simulink model "sampleModel168"  (R2021b)
settings: Solver=VariableStepAuto  StartTime=0.0  StopTime=10.0  RelTol=1e-3
undefined symbols (not defined in the file or in its folder): DiscIntNeverNeededParam
libraries: simulink x10, slpidlib x2
settings Model: Creator=user  LastModifiedBy=user

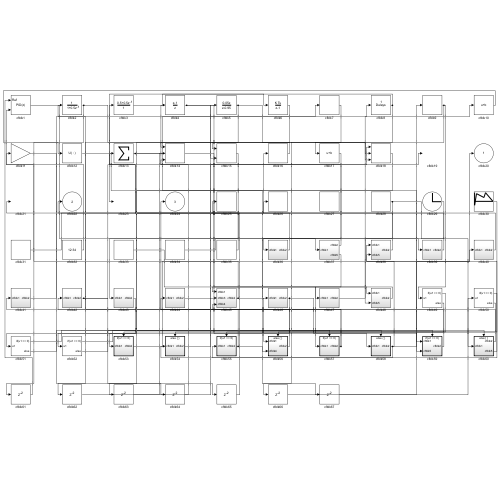
[thumbnail: Simulink's stored preview of the top-level diagram]
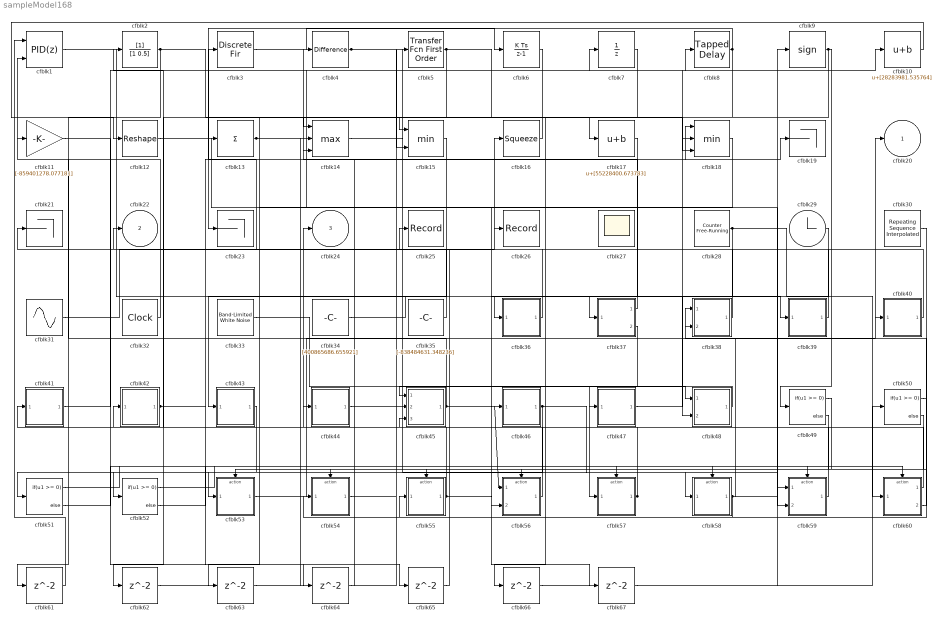
== system sampleModel168 ==
  cfblk1 : slpidlib/PID Controller (2DOF)  Controller=PID  Form=Parallel  TimeDomain=Discrete-time  UseExternalTs=off  SampleTime=1  IntegratorMethod=Forward Euler  FilterMethod=Forward Euler  ControllerParametersSource=internal  P=1  I=1  D=0  UseFilter=on  N=100  b=1  c=1  TunerSelectOption=Transfer Function Based (PID Tuner App)  InitialConditionSource=internal  InitialConditionForIntegrator=0  InitialConditionForFilter=0  DifferentiatorICPrevScaledInput=0  ExternalReset=none  TrackingMode=off  Kt=1  LimitOutput=off  SatLimitsSource=internal  UpperSaturationLimit=inf  LowerSaturationLimit=-inf  LinearizeAsGain=off  AntiWindupMode=none  Kb=1  POutMin=[]  POutMax=[]  IOutMin=[]  IOutMax=[]  DOutMin=[]  DOutMax=[]  NOutMin=[]  NOutMax=[]  bOutMin=[]  bOutMax=[]  cOutMin=[]  cOutMax=[]  SumOutMin=[]  SumOutMax=[]  SaturationOutMin=[]  SaturationOutMax=[]  PParamMin=[]  PParamMax=[]  IParamMin=[]  IParamMax=[]  DParamMin=[]  DParamMax=[]  NParamMin=[]  NParamMax=[]  bParamMin=[]  bParamMax=[]  cParamMin=[]  cParamMax=[]  KbParamMin=[]  KbParamMax=[]  KtParamMin=[]  KtParamMax=[]  KbOutMin=[]  KbOutMax=[]  KtOutMin=[]  KtOutMax=[]  IntegratorOutMin=[]  IntegratorOutMax=[]  FilterOutMin=[]  FilterOutMax=[]  SumI1OutMin=[]  SumI1OutMax=[]  SumI2OutMin=[]  SumI2OutMax=[]  SumI3OutMin=[]  SumI3OutMax=[]  SumI4OutMin=[]  SumI4OutMax=[]  SumDOutMin=[]  SumDOutMax=[]  Sum1OutMin=[]  Sum1OutMax=[]  Sum2OutMin=[]  Sum2OutMax=[]  Sum3OutMin=[]  Sum3OutMax=[]  DifferentiatorOutMin=[]  DifferentiatorOutMax=[]  FilterDiffOutCoefMin=[]  FilterDiffOutCoefMax=[]  ReciprocalOutMin=[]  ReciprocalOutMax=[]  SumDenOutMin=[]  SumDenOutMax=[]  SumNumOutMin=[]  SumNumOutMax=[]  DivideOutMin=[]  DivideOutMax=[]  UdiffTsProdOutMin=[]  UdiffTsProdOutMax=[]  NTsProdOutMin=[]  NTsProdOutMax=[]  UintegralTsProdOutMin=[]  UintegralTsProdOutMax=[]  UngainTsProdOutMin=[]  UngainTsProdOutMax=[]  IntegratorContinuousStateAttributes=''  IntegratorStateMustResolveToSignalObject=off  IntegratorRTWStateStorageClass=Auto  FilterContinuousStateAttributes=''  FilterStateMustResolveToSignalObject=off  FilterRTWStateStorageClass=Auto  ParallelPVariant=InternalParameters  IdealPVariant=Disabled  IVariant=InternalParameters  DVariant=InternalParameters  bVariant=InternalParameters  cVariant=InternalParameters  IntegratorVariant=Discrete  SatVariant=Disabled  AWVariant=Passthrough  PCopyVariant=Disabled  TRVariant=Disabled  FdbkBlocksVariant=Forward  IdealPFdbkVariant=Disabled  SatFdbkVariant=Disabled  DerivativeFilterVariant=ForwardEulerFilter  NVariant=InternalParameters  NCopyVariant=Disabled  FilterICVariant=InternalICsFilter  IntegratorICVariant=InternalICs  ExternalResetVariant=Disabled  TRSumVariant=Passthrough  SumFdbkVariant=Disabled  SumVariant=Sum_PID  TsampFilterVariant=InternalTs  TsampNgainVariant=Passthrough  TsampIntegralVariant=Passthrough  ExternalSaturationOutDataTypeStr=Inherit: Same as second input
      settings: SourceProductBaseCode=SL
  cfblk10 : Bias  Bias=[28283981.535764]
  cfblk11 : Gain  Gain=[-859401278.077181]
  cfblk12 : Reshape
  cfblk13 : Sum  Inputs=+
  cfblk14 : MinMax  Function=max  Inputs=3
  cfblk15 : MinMax  Inputs=2
  cfblk16 : Squeeze
  cfblk17 : Bias  Bias=[55228400.673783]
  cfblk18 : MinMax  Inputs=3
  cfblk19 : Terminator
  cfblk2 : DiscreteFilter  SampleTime=1
  cfblk21 : Terminator
  cfblk23 : Terminator
  cfblk25 : Record  FileSettingsInternal="{\"entries\":[{\"content\":{\"excelSettings\":{\"content\":{},\"type\":\"Streamout.ExcelSettings\"}},\"type\":\"Streamout.FileSettingStorage\",\"uuid\":\"5d6700eb-b7dc-4e89-8cfd-a7cfabde85fd\"}],\"packageUris\":[\"http://schema.mathworks.com/mf0/streamout_blocks/R2020a\"],\"version\":\"1.0\"}"  SignalsInternal="{\"entries\":[{\"content\":{\"signals\":[{\"content\":{\"blockPath\":[\"sampleModel168/cfblk25\"],\"channel\":[],\"dimensions\":[1],\"domain\":\"sampleModel168/cfblk25\",\"lineColor\":\"#ff13a6\",\"plots\":[1],\"port\":1,\"sid\":[\"\"],\"signalID\":6325,\"signalName\":\"cfblk57\"},\"type\":\"RecordBlkView.Signal\",\"uuid\":\"5bee3f64-e3fd-44b3-9e31-3812ad4f074b\"}]},\"type\":\"RecordBlkView.InputSignals\",\"uuid\":\"565ec13a-f817-448c-bf93-5228326c90da\"}],\"packageUris\":[\"http://schema.mathworks.com/mf0/streamout_blocks/R2020a\"],\"version\":\"1.0\"}"  VisualizationBindings="{\"sparklinesplugin\":{\"info\":[{\"bindingParametersList\":[],\"subplotID\":1}]}}"
  cfblk26 : Record  FileSettingsInternal="{\"entries\":[{\"content\":{\"excelSettings\":{\"content\":{},\"type\":\"Streamout.ExcelSettings\"}},\"type\":\"Streamout.FileSettingStorage\",\"uuid\":\"034f7d33-27da-4be1-a58b-e2f12ee0a9b7\"}],\"packageUris\":[\"http://schema.mathworks.com/mf0/streamout_blocks/R2020a\"],\"version\":\"1.0\"}"  SignalsInternal="{\"entries\":[{\"content\":{\"signals\":[{\"content\":{\"blockPath\":[\"sampleModel168/cfblk26\"],\"channel\":[],\"dimensions\":[1],\"domain\":\"sampleModel168/cfblk26\",\"lineColor\":\"#fe330a\",\"plots\":[1],\"port\":1,\"sid\":[\"\"],\"signalID\":6329,\"signalName\":\"cfblk31\"},\"type\":\"RecordBlkView.Signal\",\"uuid\":\"832ba97a-a374-4f23-ac50-8a6ca30bdff1\"}]},\"type\":\"RecordBlkView.InputSignals\",\"uuid\":\"b795735d-caf7-44f9-b6f9-1499413fef97\"}],\"packageUris\":[\"http://schema.mathworks.com/mf0/streamout_blocks/R2020a\"],\"version\":\"1.0\"}"  VisualizationBindings="{\"sparklinesplugin\":{\"info\":[{\"bindingParametersList\":[],\"subplotID\":1}]}}"
  cfblk27 : Scope
      settings: Floating=on
  cfblk28 : simulink/Sources/Counter Free-Running  NumBits=[13.000000]  tsamp=-1
  cfblk29 : Clock
  cfblk3 : DiscreteFir  SampleTime=1
  cfblk30 : simulink/Sources/Repeating Sequence Interpolated  OutValues=[-245595446.303233, 532111753.343580, 271370774.628076, 605929342.259745, 14003262.711225]  TimeValues=[0 0.1 0.5 0.6 1].'  LookUpMeth=Interpolation-Use End Values  tsamp=0.01  OutMin=[]  OutMax=[]  OutDataTypeStr=double  OutputDataTypeScalingMode=double  OutDataType=fixdt(0,8)  OutScaling=2^-10
  cfblk31 : Sin  Amplitude=[-188151696.405672]  Bias=[-383980109.260124]  SampleTime=0
  cfblk32 : DigitalClock
  cfblk33 : simulink/Sources/Band-Limited White Noise  Cov=[8926345468.360197]  Ts=0.1  seed=[3976395025.000000]
  cfblk34 : Constant  Value=[400865686.655921]  SampleTime=1
  cfblk35 : Constant  Value=[-838484631.348236]  SampleTime=1
  cfblk36 : Subsystem
  cfblk37 : Subsystem
  cfblk38 : Subsystem
  cfblk39 : Subsystem
  cfblk4 : simulink/Discrete/Difference  ICPrevInput=0.0  OutMin=[]  OutMax=[]  OutDataTypeStr=Inherit: Inherit via back propagation  OutDataType=fixdt(1, 16)  OutScaling=2^-10  DoSatur=off
  cfblk40 : Subsystem
  cfblk41 : Subsystem
  cfblk42 : Subsystem
  cfblk43 : Subsystem
  cfblk44 : Subsystem
  cfblk45 : Subsystem
  cfblk46 : Subsystem
  cfblk47 : Subsystem
  cfblk48 : Subsystem
  cfblk{49..52} (4 alike) : If  IfExpression=u1 >= 0  SampleTime=1
  cfblk5 : simulink/Discrete/Transfer Fcn First Order  PoleZ=0.95  ICPrevOutput=0.0  DoSatur=off
  cfblk53 : Subsystem  TreatAsAtomicUnit=on
  cfblk54 : Subsystem  TreatAsAtomicUnit=on
  cfblk55 : Subsystem  TreatAsAtomicUnit=on
  cfblk56 : Subsystem  TreatAsAtomicUnit=on
  cfblk57 : Subsystem  TreatAsAtomicUnit=on
  cfblk58 : Subsystem  TreatAsAtomicUnit=on
  cfblk59 : Subsystem  TreatAsAtomicUnit=on
  cfblk6 : DiscreteIntegrator  ICPrevOutput=DiscIntNeverNeededParam  ICPrevScaledInput=DiscIntNeverNeededParam
  cfblk60 : Subsystem  TreatAsAtomicUnit=on
  cfblk{61..67} (7 alike) : Delay  SampleTime=1
  cfblk7 : UnitDelay  HasFrameUpgradeWarning=on
  cfblk8 : simulink/Discrete/Tapped Delay  vinit=0.0  samptime=-1  NumDelays=1  DelayOrder=Oldest  includeCurrent=off
  cfblk9 : Signum
  cfblk20 : Outport
  cfblk22 : Outport  Port=2
  cfblk24 : Outport  Port=3
  wires:
  cfblk39/1(cfblk2) -> cfblk16/1
  cfblk2/1 -> cfblk15/2, cfblk61/1
  cfblk53/1(cfblk2) -> cfblk20/1
  cfblk1/1 -> cfblk39/1(cfblk1)
  cfblk55/1(cfblk2) -> cfblk44/1(cfblk1), cfblk67/1
  cfblk14/1 -> cfblk48/1(cfblk1)
  cfblk4/1 -> cfblk58/1(cfblk1), cfblk18/3
  cfblk10/1 -> cfblk12/1
  cfblk8/1 -> cfblk23/1, cfblk63/1
  cfblk29/1 -> cfblk48/2(cfblk5)
  cfblk9/1 -> cfblk49/1, cfblk17/1
  cfblk31/1 -> cfblk26/1
  cfblk43/1(cfblk2) -> cfblk51/1
  cfblk48/1(cfblk2) -> cfblk45/1(cfblk1)
  cfblk30/1 -> cfblk55/1(cfblk1)
  cfblk46/1(cfblk2) -> cfblk52/1, cfblk59/2(cfblk5)
  cfblk34/1 -> cfblk37/1(cfblk1)
  cfblk59/1(cfblk2) -> cfblk42/1(cfblk1)
  cfblk45/1(cfblk2) -> cfblk56/1(cfblk1), cfblk11/1
  cfblk15/1 -> cfblk43/1(cfblk1)
  cfblk12/1 -> cfblk46/1(cfblk1)
  cfblk28/1 -> cfblk56/2(cfblk4), cfblk60/1(cfblk1)
  cfblk44/1(cfblk2) -> cfblk5/1
  cfblk38/1(cfblk2) -> cfblk3/1
  cfblk7/1 -> cfblk36/1(cfblk1)
  cfblk60/1(cfblk2) -> cfblk24/1
  cfblk3/1 -> cfblk6/1
  cfblk32/1 -> cfblk1/2
  cfblk60/2(cfblk5) -> cfblk38/1(cfblk1)
  cfblk40/1(cfblk2) -> cfblk13/1
  cfblk36/1(cfblk2) -> cfblk22/1
  cfblk13/1 -> cfblk8/1, cfblk59/1(cfblk1)
  cfblk35/1 -> cfblk21/1
  cfblk54/1(cfblk2) -> cfblk19/1
  cfblk42/1(cfblk2) -> cfblk18/1, cfblk64/1
  cfblk18/1 -> cfblk53/1(cfblk1)
  cfblk58/1(cfblk2) -> cfblk38/2(cfblk5), cfblk40/1(cfblk1), cfblk54/1(cfblk1)
  cfblk37/1(cfblk2) -> cfblk4/1
  cfblk33/1 -> cfblk57/1(cfblk1)
  cfblk57/1(cfblk2) -> cfblk25/1, cfblk41/1(cfblk1)
  cfblk41/1(cfblk2) -> cfblk7/1
  cfblk16/1 -> cfblk14/1
  cfblk56/1(cfblk2) -> cfblk2/1
  cfblk37/2(cfblk5) -> cfblk47/1(cfblk1)
  cfblk47/1(cfblk2) -> cfblk10/1
  cfblk5/1 -> cfblk18/2, cfblk15/1
  cfblk49/1 -> cfblk53/Action
  cfblk49/2 -> cfblk54/Action
  cfblk50/1 -> cfblk55/Action
  cfblk50/2 -> cfblk56/Action
  cfblk51/1 -> cfblk57/Action
  cfblk51/2 -> cfblk58/Action
  cfblk52/1 -> cfblk59/Action
  cfblk52/2 -> cfblk60/Action
  cfblk61/1 -> cfblk1/1
  cfblk6/1 -> cfblk62/1
  cfblk62/1 -> cfblk45/2(cfblk3)
  cfblk63/1 -> cfblk14/2
  cfblk64/1 -> cfblk14/3
  cfblk11/1 -> cfblk65/1
  cfblk65/1 -> cfblk45/3(cfblk4)
  cfblk17/1 -> cfblk66/1
  cfblk66/1 -> cfblk9/1
  cfblk67/1 -> cfblk50/1

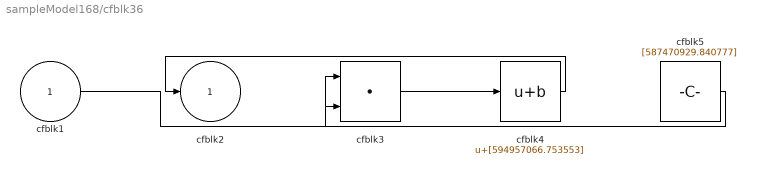
== system sampleModel168/cfblk36 ==
  cfblk1 : Inport
  cfblk3 : DotProduct  InputSameDT=on  OutDataTypeStr=Inherit: Inherit via internal rule
  cfblk4 : Bias  Bias=[594957066.753553]
  cfblk5 : Constant  Value=[587470929.840777]  SampleTime=1
  cfblk2 : Outport
  wires:
  cfblk4/1 -> cfblk2/1
  cfblk5/1 -> cfblk3/1
  cfblk1/1 -> cfblk3/2
  cfblk3/1 -> cfblk4/1

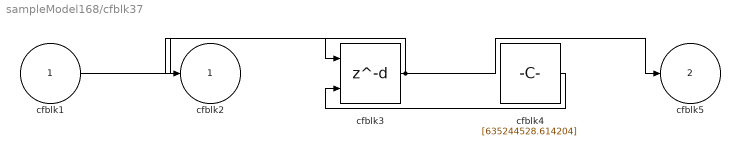
== system sampleModel168/cfblk37 ==
  cfblk1 : Inport
  cfblk3 : Delay  DelayLengthSource=Input port  SampleTime=1
      settings: InputPortMap=u0,p1
  cfblk4 : Constant  Value=[635244528.614204]  SampleTime=1
  cfblk2 : Outport
  cfblk5 : Outport  Port=2
  wires:
  cfblk1/1 -> cfblk3/1
  cfblk4/1 -> cfblk3/2
  cfblk3/1 -> cfblk5/1, cfblk2/1

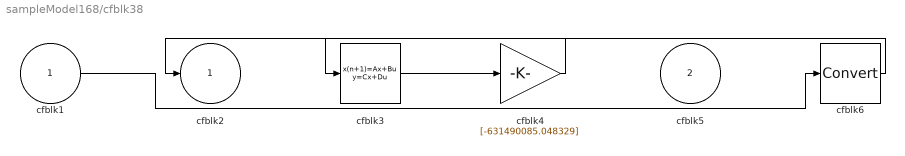
== system sampleModel168/cfblk38 ==
  cfblk1 : Inport
  cfblk5 : Inport  Port=2
  cfblk3 : DiscreteStateSpace
  cfblk4 : Gain  Gain=[-631490085.048329]
  cfblk6 : DataTypeConversion
  cfblk2 : Outport
  wires:
  cfblk4/1 -> cfblk2/1
  cfblk3/1 -> cfblk4/1
  cfblk1/1 -> cfblk6/1
  cfblk6/1 -> cfblk3/1

== system sampleModel168/cfblk39 ==
  cfblk1 : Inport
  cfblk3 : Delay  ShowEnablePort=on  SampleTime=1
      settings: InputPortMap=u0,e6
  cfblk4 : Product  Inputs=*
  cfblk2 : Outport
  wires:
  cfblk3/1 -> cfblk4/1
  cfblk4/1 -> cfblk2/1
  cfblk1/1 -> cfblk3/1, cfblk3/2

== system sampleModel168/cfblk40 ==
  cfblk1 : Inport
  cfblk3 : Assignment  DiagnosticForDimensions=Warning  IndexOptions=Index vector (dialog)  Indices=1  OutputSizes=1
  cfblk4 : Squeeze
  cfblk5 : Delay  SampleTime=1
  cfblk2 : Outport
  wires:
  cfblk1/1 -> cfblk2/1, cfblk3/2
  cfblk3/1 -> cfblk4/1
  cfblk4/1 -> cfblk5/1
  cfblk5/1 -> cfblk3/1

== system sampleModel168/cfblk41 ==
  cfblk1 : Inport
  cfblk3 : Constant  Value=[481463606.367237]  SampleTime=1
  cfblk2 : Outport
  wires:
  cfblk1/1 -> cfblk2/1

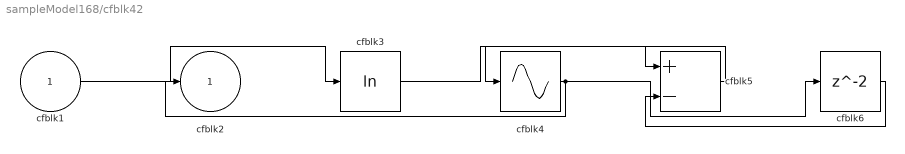
== system sampleModel168/cfblk42 ==
  cfblk1 : Inport
  cfblk3 : Math  Operator=log  SaturateOnIntegerOverflow=on
  cfblk4 : Sin  TimeSource=Use external signal  SampleTime=0
  cfblk5 : Sum  Inputs=+-
  cfblk6 : Delay  SampleTime=1
  cfblk2 : Outport
  wires:
  cfblk5/1 -> cfblk4/1
  cfblk1/1 -> cfblk3/1
  cfblk4/1 -> cfblk2/1, cfblk6/1
  cfblk3/1 -> cfblk5/1
  cfblk6/1 -> cfblk5/2

== system sampleModel168/cfblk43 ==
  cfblk1 : Inport
  cfblk3 : Sum
  cfblk4 : Sqrt  SaturateOnIntegerOverflow=on
  cfblk2 : Outport
  wires:
  cfblk4/1 -> cfblk2/1
  cfblk1/1 -> cfblk3/1, cfblk3/2
  cfblk3/1 -> cfblk4/1

== system sampleModel168/cfblk44 ==
  cfblk1 : Inport
  cfblk3 : DiscreteFilter  SampleTime=1
  cfblk2 : Outport
  wires:
  cfblk3/1 -> cfblk2/1
  cfblk1/1 -> cfblk3/1

== system sampleModel168/cfblk45 ==
  cfblk1 : Inport
  cfblk3 : Inport  Port=2
  cfblk4 : Inport  Port=3
  cfblk2 : Outport
  wires:
  cfblk3/1 -> cfblk2/1

== system sampleModel168/cfblk46 ==
  cfblk1 : Inport
  cfblk3 : Sum  Inputs=+-
  cfblk4 : Constant  Value=[-620973780.645703]  SampleTime=1
  cfblk2 : Outport
  wires:
  cfblk4/1 -> cfblk3/1
  cfblk1/1 -> cfblk3/2
  cfblk3/1 -> cfblk2/1

== system sampleModel168/cfblk47 ==
  cfblk1 : Inport
  cfblk3 : simulink/Discrete/Transfer Fcn Real Zero  ZeroZ=0.75  ICPrevInput=0.0  DoSatur=off
      settings: SourceProductBaseCode=SL
  cfblk4 : simulink/Discrete/Transfer Fcn Lead or Lag  PoleZ=0.95  ZeroZ=0.75  ICPrevOutput=0.0  ICPrevInput=0.0  DoSatur=off
      settings: SourceProductBaseCode=SL
  cfblk5 : simulink/Discrete/Transfer Fcn First Order  PoleZ=0.95  ICPrevOutput=0.0  DoSatur=off
  cfblk2 : Outport
  wires:
  cfblk1/1 -> cfblk5/1, cfblk3/1
  cfblk4/1 -> cfblk2/1
  cfblk5/1 -> cfblk4/1

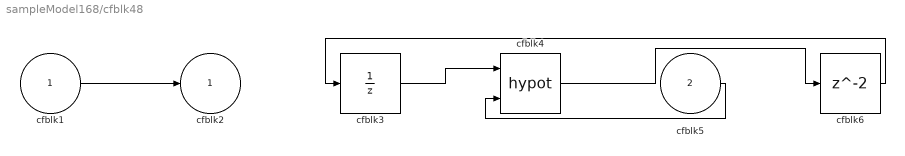
== system sampleModel168/cfblk48 ==
  cfblk1 : Inport
  cfblk5 : Inport  Port=2
  cfblk3 : UnitDelay  HasFrameUpgradeWarning=on
  cfblk4 : Math  Operator=hypot  SaturateOnIntegerOverflow=on
  cfblk6 : Delay  SampleTime=1
  cfblk2 : Outport
  wires:
  cfblk3/1 -> cfblk4/1
  cfblk1/1 -> cfblk2/1
  cfblk5/1 -> cfblk4/2
  cfblk4/1 -> cfblk6/1
  cfblk6/1 -> cfblk3/1

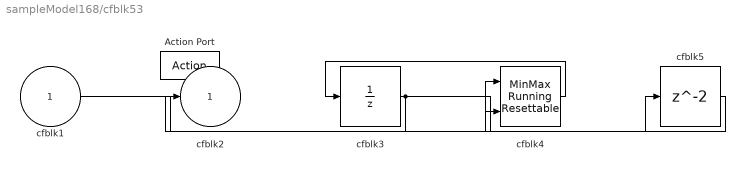
== system sampleModel168/cfblk53 ==
  cfblk1 : Inport
  Action Port : ActionPort  ActionPortLabel=if(u1 >= 0)
  cfblk3 : UnitDelay  SampleTime=-1  HasFrameUpgradeWarning=on
  cfblk4 : simulink/Math Operations/MinMax Running Resettable  Function=min  vinit=0.0
  cfblk5 : Delay
  cfblk2 : Outport
  wires:
  cfblk1/1 -> cfblk4/1
  cfblk4/1 -> cfblk3/1
  cfblk3/1 -> cfblk2/1, cfblk5/1
  cfblk5/1 -> cfblk4/2

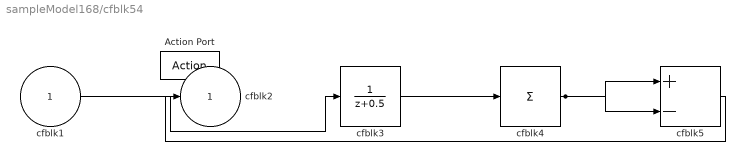
== system sampleModel168/cfblk54 ==
  cfblk1 : Inport
  Action Port : ActionPort  ActionPortLabel=else
  cfblk3 : DiscreteTransferFcn
  cfblk4 : Sum  Inputs=+
  cfblk5 : Sum  Inputs=+-
  cfblk2 : Outport
  wires:
  cfblk1/1 -> cfblk3/1
  cfblk5/1 -> cfblk2/1
  cfblk3/1 -> cfblk4/1
  cfblk4/1 -> cfblk5/1, cfblk5/2

== system sampleModel168/cfblk55 ==
  cfblk1 : Inport
  Action Port : ActionPort  ActionPortLabel=if(u1 >= 0)
  cfblk3 : Constant  Value=[634847590.051330]  SampleTime=1
  cfblk2 : Outport
  wires:
  cfblk1/1 -> cfblk2/1

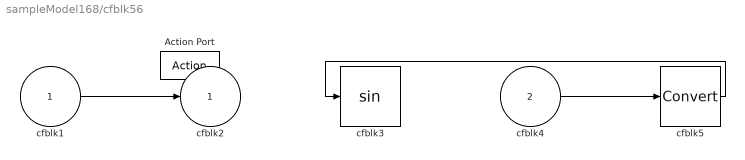
== system sampleModel168/cfblk56 ==
  cfblk1 : Inport
  cfblk4 : Inport  Port=2
  Action Port : ActionPort  ActionPortLabel=else
  cfblk3 : Trigonometry
  cfblk5 : DataTypeConversion
  cfblk2 : Outport
  wires:
  cfblk1/1 -> cfblk2/1
  cfblk4/1 -> cfblk5/1
  cfblk5/1 -> cfblk3/1

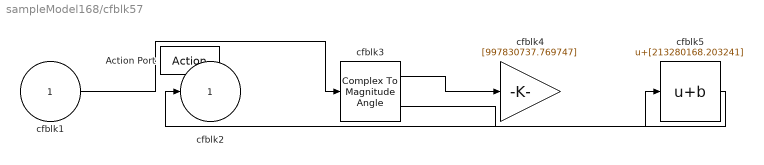
== system sampleModel168/cfblk57 ==
  cfblk1 : Inport
  Action Port : ActionPort  ActionPortLabel=if(u1 >= 0)
  cfblk3 : ComplexToMagnitudeAngle
  cfblk4 : Gain  Gain=[997830737.769747]
  cfblk5 : Bias  Bias=[213280168.203241]
  cfblk2 : Outport
  wires:
  cfblk5/1 -> cfblk2/1
  cfblk3/1 -> cfblk4/1
  cfblk3/2 -> cfblk5/1
  cfblk1/1 -> cfblk3/1

== system sampleModel168/cfblk58 ==
  cfblk1 : Inport
  Action Port : ActionPort  ActionPortLabel=else
  cfblk3 : slpidlib/PID Controller (2DOF)  Controller=PID  Form=Parallel  TimeDomain=Discrete-time  UseExternalTs=off  SampleTime=-1  IntegratorMethod=Forward Euler  FilterMethod=Forward Euler  ControllerParametersSource=internal  P=1  I=1  D=0  UseFilter=on  N=100  b=1  c=1  TunerSelectOption=Transfer Function Based (PID Tuner App)  InitialConditionSource=internal  InitialConditionForIntegrator=0  InitialConditionForFilter=0  DifferentiatorICPrevScaledInput=0  ExternalReset=none  TrackingMode=off  Kt=1  LimitOutput=off  SatLimitsSource=internal  UpperSaturationLimit=inf  LowerSaturationLimit=-inf  LinearizeAsGain=off  AntiWindupMode=none  Kb=1  POutMin=[]  POutMax=[]  IOutMin=[]  IOutMax=[]  DOutMin=[]  DOutMax=[]  NOutMin=[]  NOutMax=[]  bOutMin=[]  bOutMax=[]  cOutMin=[]  cOutMax=[]  SumOutMin=[]  SumOutMax=[]  SaturationOutMin=[]  SaturationOutMax=[]  PParamMin=[]  PParamMax=[]  IParamMin=[]  IParamMax=[]  DParamMin=[]  DParamMax=[]  NParamMin=[]  NParamMax=[]  bParamMin=[]  bParamMax=[]  cParamMin=[]  cParamMax=[]  KbParamMin=[]  KbParamMax=[]  KtParamMin=[]  KtParamMax=[]  KbOutMin=[]  KbOutMax=[]  KtOutMin=[]  KtOutMax=[]  IntegratorOutMin=[]  IntegratorOutMax=[]  FilterOutMin=[]  FilterOutMax=[]  SumI1OutMin=[]  SumI1OutMax=[]  SumI2OutMin=[]  SumI2OutMax=[]  SumI3OutMin=[]  SumI3OutMax=[]  SumI4OutMin=[]  SumI4OutMax=[]  SumDOutMin=[]  SumDOutMax=[]  Sum1OutMin=[]  Sum1OutMax=[]  Sum2OutMin=[]  Sum2OutMax=[]  Sum3OutMin=[]  Sum3OutMax=[]  DifferentiatorOutMin=[]  DifferentiatorOutMax=[]  FilterDiffOutCoefMin=[]  FilterDiffOutCoefMax=[]  ReciprocalOutMin=[]  ReciprocalOutMax=[]  SumDenOutMin=[]  SumDenOutMax=[]  SumNumOutMin=[]  SumNumOutMax=[]  DivideOutMin=[]  DivideOutMax=[]  UdiffTsProdOutMin=[]  UdiffTsProdOutMax=[]  NTsProdOutMin=[]  NTsProdOutMax=[]  UintegralTsProdOutMin=[]  UintegralTsProdOutMax=[]  UngainTsProdOutMin=[]  UngainTsProdOutMax=[]  IntegratorContinuousStateAttributes=''  IntegratorStateMustResolveToSignalObject=off  IntegratorRTWStateStorageClass=Auto  FilterContinuousStateAttributes=''  FilterStateMustResolveToSignalObject=off  FilterRTWStateStorageClass=Auto  ParallelPVariant=InternalParameters  IdealPVariant=Disabled  IVariant=InternalParameters  DVariant=InternalParameters  bVariant=InternalParameters  cVariant=InternalParameters  IntegratorVariant=Discrete  SatVariant=Disabled  AWVariant=Passthrough  PCopyVariant=Disabled  TRVariant=Disabled  FdbkBlocksVariant=Forward  IdealPFdbkVariant=Disabled  SatFdbkVariant=Disabled  DerivativeFilterVariant=ForwardEulerFilter  NVariant=InternalParameters  NCopyVariant=Disabled  FilterICVariant=InternalICsFilter  IntegratorICVariant=InternalICs  ExternalResetVariant=Disabled  TRSumVariant=Passthrough  SumFdbkVariant=Disabled  SumVariant=Sum_PID  TsampFilterVariant=InternalTs  TsampNgainVariant=Passthrough  TsampIntegralVariant=Passthrough  ExternalSaturationOutDataTypeStr=Inherit: Same as second input
      settings: SourceProductBaseCode=SL
  cfblk2 : Outport
  wires:
  cfblk1/1 -> cfblk3/1, cfblk3/2
  cfblk3/1 -> cfblk2/1

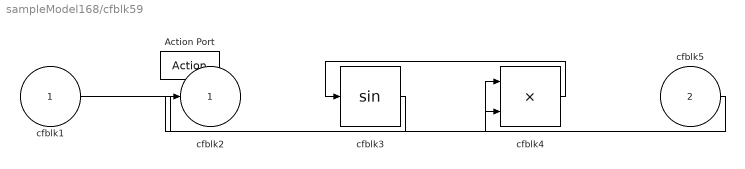
== system sampleModel168/cfblk59 ==
  cfblk1 : Inport
  cfblk5 : Inport  Port=2
  Action Port : ActionPort  ActionPortLabel=if(u1 >= 0)
  cfblk3 : Trigonometry
  cfblk4 : Product
  cfblk2 : Outport
  wires:
  cfblk4/1 -> cfblk3/1
  cfblk1/1 -> cfblk4/1
  cfblk3/1 -> cfblk2/1
  cfblk5/1 -> cfblk4/2

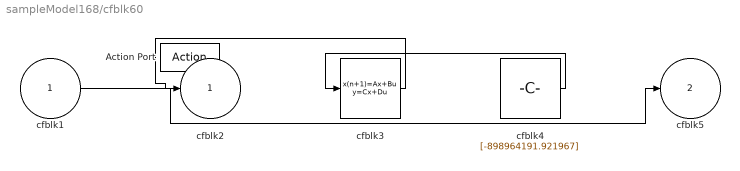
== system sampleModel168/cfblk60 ==
  cfblk1 : Inport
  Action Port : ActionPort  ActionPortLabel=else
  cfblk3 : DiscreteStateSpace  SampleTime=-1
  cfblk4 : Constant  Value=[-898964191.921967]  SampleTime=1
  cfblk2 : Outport
  cfblk5 : Outport  Port=2
  wires:
  cfblk1/1 -> cfblk5/1
  cfblk3/1 -> cfblk2/1
  cfblk4/1 -> cfblk3/1
